simulink model "Point71_simulink_z"  (R2024b)
settings: Solver=VariableStepAuto  StartTime=0.0  StopTime=tsim  RelTol=1e-3
undefined symbols (not defined in the file): Ad, B_noise, Bd, Cd, D_noise, Dd, Discrete, du_max, du_min, input, N, NK, Pr, Q_LQ, R_LQ, RK, Time, Ts, U_bar_dis, u_prev, umax, umin, x, x0, xmax, xmin, xref, ZahraMPC7_vel
libraries: simulink x2, ctrlSharedLib x1
settings Model: Creator=zalem  LastModifiedBy=zalem

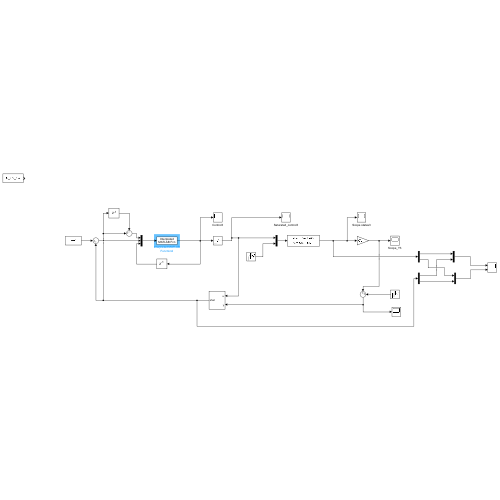
[thumbnail: Simulink's stored preview of the top-level diagram]
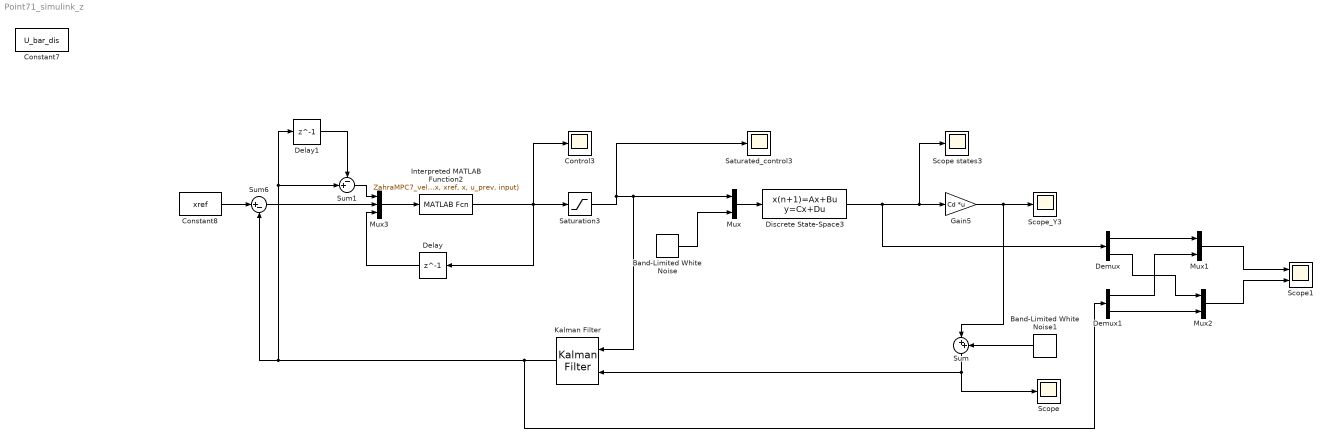
== system Point71_simulink_z ==
  Band-Limited White Noise : simulink/Sources/Band-Limited White Noise  Cov=power_vx  Ts=Ts  seed=[23341]
  Band-Limited White Noise1 : simulink/Sources/Band-Limited White Noise  Cov=power_vy  Ts=Ts  seed=[23341]
  Constant7 : Constant  Value=U_bar_dis
  Constant8 : Constant  Value=xref
  Control3 : Scope
  Delay : Delay  DelayLength=1
  Delay1 : Delay  DelayLength=1
  Demux : Demux  Outputs=2
  Demux1 : Demux  Outputs=2
  Discrete State-Space3 : DiscreteStateSpace  A=Ad  B=B_noise  C=Cd  D=D_noise  InitialCondition=x0  SampleTime=Ts
  Gain5 : Gain  Gain=Cd  Multiplication=Matrix(K*u)
  Interpreted MATLAB Function2 : MATLABFcn  MATLABFcn=ZahraMPC7_vel(Ad, Bd, Q_LQ, R_LQ, Pr, N, du_min, du_max, umin, umax, U_bar_dis, xmin, xmax, xref, x, u_prev, input)  OutputDimensions=2
  Kalman Filter : ctrlSharedLib/Kalman Filter  TimeDomain=Discrete-Time  UseCurrentEstimator=on  ModelSource=Individual A, B, C, D matrices  ModelSourceVariable=ss(0.95,1,1,0,1)  A=Ad  B=Bd  C=Cd  D=Dd  NumberOfStates=1  NumberOfInputs=1  NumberOfOutputs=1  InitialEstimateSource=Dialog  X0=0  P0=10  UseK=off  UseGH=off  NumberOfProcessNoiseInputs=1  G=1  TimeInvariantG=on  H=0  TimeInvariantH=on  Q=QK  TimeInvariantQ=on  R=RK  TimeInvariantR=on  N=NK  TimeInvariantN=on  AddInputPort=on  AddEnablePort=off  OutputEstimatedY=off  OutputP=off  Ts=-1
  Mux : Mux  Inputs=2
  Mux1 : Mux  Inputs=2
  Mux2 : Mux  Inputs=2
  Mux3 : Mux  Inputs=3
  Saturated_control3 : Scope
  Saturation3 : Saturate  UpperLimit=inf  LowerLimit=-inf
  Scope : Scope
  Scope states3 : Scope
  Scope1 : Scope  NumInputPorts=2
  Scope_Y3 : Scope
  Sum : Sum  Inputs=|++
  Sum1 : Sum  Inputs=-+|
  Sum6 : Sum  Inputs=|+-
  wires:
  Discrete State-Space3/1 -> Demux/1, Gain5/1, Scope states3/1
  Constant8/1 -> Sum6/1
  Interpreted MATLAB Function2/1 -> Delay/1, Control3/1, Saturation3/1
  Gain5/1 -> Sum/1, Scope_Y3/1
  Saturation3/1 -> Saturated_control3/1, Kalman Filter/1, Mux/1
  Mux/1 -> Discrete State-Space3/1
  Band-Limited White Noise/1 -> Mux/2
  Kalman Filter/1 -> Demux1/1, Delay1/1, Sum1/2, Sum6/2
  Band-Limited White Noise1/1 -> Sum/2
  Sum/1 -> Scope/1, Kalman Filter/2
  Mux1/1 -> Scope1/1
  Demux/1 -> Mux1/1
  Demux1/2 -> Mux2/2
  Demux1/1 -> Mux1/2
  Demux/2 -> Mux2/1
  Mux2/1 -> Scope1/2
  Delay/1 -> Mux3/3
  Sum6/1 -> Mux3/2
  Delay1/1 -> Sum1/1
  Sum1/1 -> Mux3/1
  Mux3/1 -> Interpreted MATLAB Function2/1
